simulink model "CanceladorEco"  (R2013a)
settings: Solver=ode45  SolverMode=SingleTasking  StartTime=0.0  StopTime=10.0  RelTol=1e-3
values from neighbouring files (symbols this model uses):
  T = 1    [Variaveis.mat]
settings Model: Creator=Afonso  LastModifiedBy=Élio
settings DataIOCC: SignalLoggingSaveFormat=ModelDataLogs
settings OptimizationCC: BlockReduction=off  BooleanDataType=off
settings DebuggingCC: SaveWithParameterizedLinksMsg=none  SignalResolutionControl=TryResolveAllWithWarning  SolverPrmCheckMsg=none  MultiTaskDSMMsg=warning  MultiTaskCondExecSysMsg=none  StrictBusMsg=None
settings HardwareCC: TargetUnknown=on
settings RTWCC: IncludeERTFirstTime=on

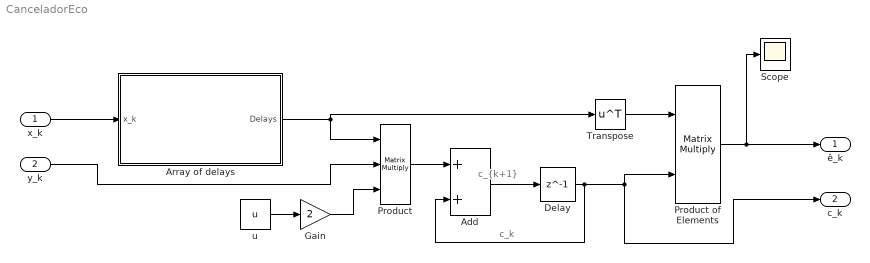
== system CanceladorEco ==
  note: c_k
  note: c_{k+1}
  x_k : Inport
  y_k : Inport  Port=2
  Add : Sum
  Array of delays : Subsystem
  Delay : Delay  DelayLength=1  SampleTime=T
  Gain : Gain  Gain=2
  Product : Product  Inputs=3  Multiplication=Matrix(*)
  Product of Elements : Product  Inputs=**  Multiplication=Matrix(*)
  Scope : Scope
  Transpose : Math  Operator=transpose  SaturateOnIntegerOverflow=on
  u : Constant  Value=u  SampleTime=T
  ê_k : Outport
  c_k : Outport  Port=2
  wires:
  y_k/1 -> Product/2
  u/1 -> Gain/1
  Gain/1 -> Product/3
  x_k/1 -> Array of delays/1(x_k)
  Product/1 -> Add/1
  Product of Elements/1 -> ê_k/1, Scope/1
  Add/1 -> Delay/1
  Delay/1 -> c_k/1, Product of Elements/2, Add/2
  Transpose/1 -> Product of Elements/1
  Array of delays/1(Delays) -> Product/1, Transpose/1

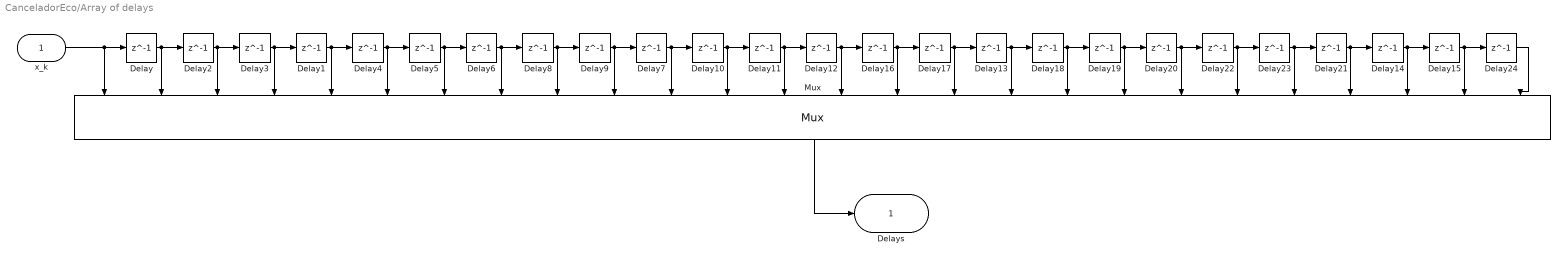
== system CanceladorEco/Array of delays ==
  x_k : Inport
  Delay : Delay  DelayLength=1  SampleTime=T
  Delay{1..24} (24 alike) : Delay  DelayLength=1
  Mux : Mux  Inputs=26
      settings: DisplayOption=signals
  Delays : Outport
  wires:
  Delay/1 -> Delay2/1, Mux/2
  Delay2/1 -> Mux/3, Delay3/1
  Delay11/1 -> Mux/13, Delay12/1
  Delay24/1 -> Mux/26
  Delay19/1 -> Delay20/1, Mux/19
  x_k/1 -> Delay/1, Mux/1
  Mux/1 -> Delays/1
  Delay15/1 -> Delay24/1, Mux/25
  Delay4/1 -> Mux/6, Delay5/1
  Delay1/1 -> Mux/5, Delay4/1
  Delay5/1 -> Mux/7, Delay6/1
  Delay12/1 -> Mux/14, Delay16/1
  Delay18/1 -> Mux/18, Delay19/1
  Delay16/1 -> Mux/15, Delay17/1
  Delay23/1 -> Delay21/1, Mux/22
  Delay17/1 -> Mux/16, Delay13/1
  Delay22/1 -> Delay23/1, Mux/21
  Delay14/1 -> Delay15/1, Mux/24
  Delay20/1 -> Delay22/1, Mux/20
  Delay13/1 -> Mux/17, Delay18/1
  Delay21/1 -> Delay14/1, Mux/23
  Delay8/1 -> Mux/9, Delay9/1
  Delay6/1 -> Mux/8, Delay8/1
  Delay10/1 -> Delay11/1, Mux/12
  Delay9/1 -> Delay7/1, Mux/10
  Delay7/1 -> Mux/11, Delay10/1
  Delay3/1 -> Mux/4, Delay1/1
